simulink model "Dreamer_3dof"  (R2023b)
settings: Solver=FixedStepAuto  StartTime=0.0  StopTime=10.0  FixedStep=.01  RelTol=1e-3
settings Model: Creator=kbs_s  LastModifiedBy=kbs_s

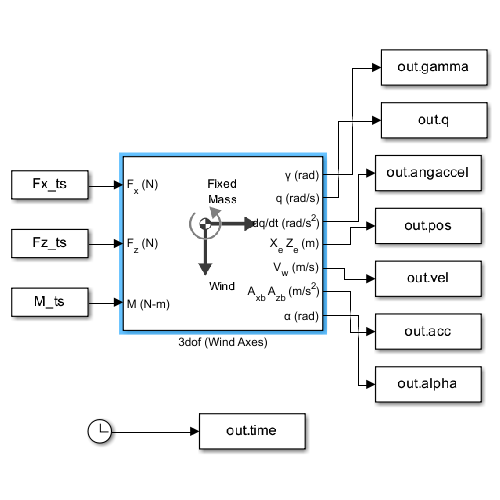
[thumbnail: Simulink's stored preview of the top-level diagram]
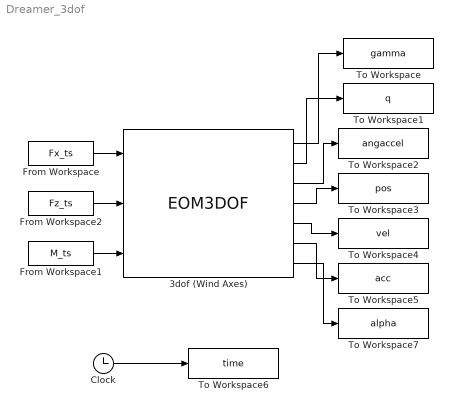
== system Dreamer_3dof ==
  3dof (Wind Axes) : EOM3DOF  axes=Wind  v_ini=1  Iyy=1
  Clock : Clock
  From Workspace : FromWorkspace  VariableName=Fx_ts
  From Workspace1 : FromWorkspace  VariableName=M_ts
  From Workspace2 : FromWorkspace  VariableName=Fz_ts
  To Workspace : ToWorkspace  VariableName=gamma  SaveFormat=Timeseries  SampleTime=-1
  To Workspace1 : ToWorkspace  VariableName=q  SaveFormat=Timeseries  SampleTime=-1
  To Workspace2 : ToWorkspace  VariableName=angaccel  SaveFormat=Timeseries  SampleTime=-1
  To Workspace3 : ToWorkspace  VariableName=pos  SaveFormat=Timeseries  SampleTime=-1
  To Workspace4 : ToWorkspace  VariableName=vel  SaveFormat=Timeseries  SampleTime=-1
  To Workspace5 : ToWorkspace  VariableName=acc  SaveFormat=Timeseries  SampleTime=-1
  To Workspace6 : ToWorkspace  VariableName=time  SampleTime=-1
  To Workspace7 : ToWorkspace  VariableName=alpha  SaveFormat=Timeseries  SampleTime=-1
  wires:
  From Workspace/1 -> 3dof (Wind Axes)/1
  From Workspace2/1 -> 3dof (Wind Axes)/2
  From Workspace1/1 -> 3dof (Wind Axes)/3
  3dof (Wind Axes)/1 -> To Workspace/1
  3dof (Wind Axes)/2 -> To Workspace1/1
  3dof (Wind Axes)/3 -> To Workspace2/1
  3dof (Wind Axes)/4 -> To Workspace3/1
  3dof (Wind Axes)/5 -> To Workspace4/1
  3dof (Wind Axes)/6 -> To Workspace5/1
  Clock/1 -> To Workspace6/1
  3dof (Wind Axes)/7 -> To Workspace7/1
